simulink model "back_calculation"  (R2023b)
settings: Solver=FixedStepAuto  StartTime=0.0  StopTime=50  FixedStep=parameters.ts  RelTol=1e-3
values from neighbouring files (symbols this model uses):
  parameters = back_calculation3(1)    [simulation1.m]    (also in simulation2.m = IntegracaoCondicional(1))
undefined symbols (not defined in the file or in its folder): DiscIntNeverNeededParam
libraries: simulink x1
settings Model: Creator=death  LastModifiedBy=death

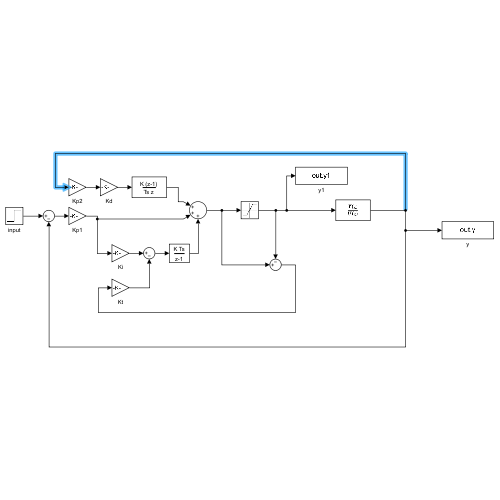
[thumbnail: Simulink's stored preview of the top-level diagram]
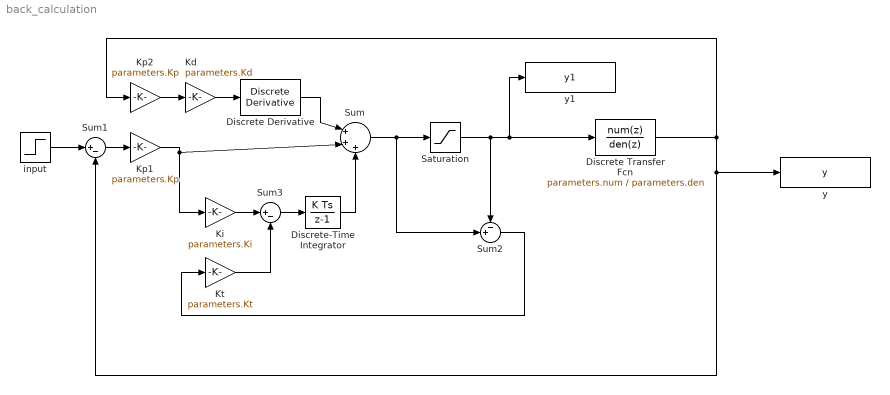
== system back_calculation ==
  Discrete Transfer Fcn : DiscreteTransferFcn  Numerator=parameters.num  Denominator=parameters.den
  Discrete Derivative : simulink/Discrete/Discrete Derivative  gainval=parameters.ts  ICPrevScaledInput=0.0  OutMin=[]  OutMax=[]  OutDataType=fixdt(1, 16)  OutScaling=2^-10  DoSatur=off
  Discrete-Time Integrator : DiscreteIntegrator  SampleTime=parameters.ts  ICPrevOutput=DiscIntNeverNeededParam  ICPrevScaledInput=DiscIntNeverNeededParam
  Kd : Gain  Gain=parameters.Kd
  Ki : Gain  Gain=parameters.Ki
  Kp1 : Gain  Gain=parameters.Kp
  Kp2 : Gain  Gain=parameters.Kp
  Kt : Gain  Gain=parameters.Kt
  Saturation : Saturate  UpperLimit=parameters.upper_limit  LowerLimit=parameters.lower_limit
  Sum : Sum  Inputs=|+++
  Sum1 : Sum  Inputs=|+-
  Sum2 : Sum  Inputs=-+|
  Sum3 : Sum  Inputs=|+-
  input : Step  Time=parameters.step_time  Before=parameters.initial_value  After=parameters.final_value  SampleTime=parameters.sample_time
  y : ToWorkspace  VariableName=y  SaveFormat=Structure With Time  SampleTime=parameters.ts
  y1 : ToWorkspace  VariableName=y1  SaveFormat=Structure With Time  SampleTime=parameters.ts
  wires:
  Discrete Transfer Fcn/1 -> Kp2/1, y/1, Sum1/2
  Kp2/1 -> Kd/1
  Kd/1 -> Discrete Derivative/1
  Saturation/1 -> Discrete Transfer Fcn/1, y1/1, Sum2/1
  Ki/1 -> Sum3/1
  Sum3/1 -> Discrete-Time Integrator/1
  Sum2/1 -> Kt/1
  Discrete-Time Integrator/1 -> Sum/3
  Discrete Derivative/1 -> Sum/1
  Kt/1 -> Sum3/2
  Kp1/1 -> Sum/2, Ki/1
  Sum1/1 -> Kp1/1
  Sum/1 -> Sum2/2, Saturation/1
  input/1 -> Sum1/1
